simulink model "feed_system_harness_combined"  (R2025b)
settings: Solver=ode23t  StartTime=0  StopTime=8  RelTol=1e-3
undefined symbols (not defined in the file): eregValveDelay, fuelMdot, fuelRho, fuelSetpoint, KcFuel, Kp1Fuel, Kp2Fuel, KpRampTimeFuel, mainValveTime, modelName, OFRatio, T_prop_n2
libraries: fl_lib x11, nesl_utility x9, simulink x4
(part 2 of 2)

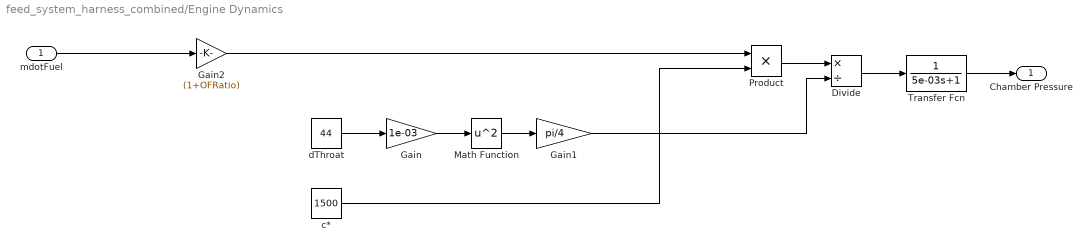
== system feed_system_harness_combined/Engine Dynamics ==
  mdotFuel : Inport
  Divide : Product  Inputs=*/
  Gain : Gain  Gain=1e-03
  Gain1 : Gain  Gain=pi/4
  Gain2 : Gain  Gain=(1+OFRatio)
  Math Function : Math  Operator=square
  Product : Product
  Transfer Fcn : TransferFcn  Denominator=[5e-03 1]
  c* : Constant  Value=1500
  dThroat : Constant  Value=44
  Chamber Pressure : Outport
  wires:
  dThroat/1 -> Gain/1
  Gain/1 -> Math Function/1
  Math Function/1 -> Gain1/1
  c*/1 -> Product/2
  Product/1 -> Divide/1
  Gain1/1 -> Divide/2
  Divide/1 -> Transfer Fcn/1
  Transfer Fcn/1 -> Chamber Pressure/1
  mdotFuel/1 -> Gain2/1
  Gain2/1 -> Product/1

== matlab function feed_system_harness_combined/FeedBack Command ==
  data: propPressure input; propSetpoint input; valveAngle output; nd_error output; Kp input
function [valveAngle, nd_error] = eregControl(propPressure, propSetpoint, Kp)
nd_error = (1 - propPressure/propSetpoint); %Non dimensional error
theta = nd_error * Kp;  %In degrees

valveAngle = deg2rad(theta);

== matlab function feed_system_harness_combined/FeedForwardCommand Fuel ==
  data: n2Pressure input; valveAngle output; CdA_measured output; CdACorrectionFactor input; CdAArray input; mdotProp input; rhoProp input; CdA output
function [valveAngle, CdA_measured, CdA] = feedForwardAngle(n2Pressure, CdACorrectionFactor, CdAArray, mdotProp, rhoProp)
    % Required effective flow area
    CdA_measured = (mdotProp / rhoProp) * 1/sqrt(max(0,n2Pressure)) * 0.673;
    CdA = CdA_measured * CdACorrectionFactor;
% Ball valve opening angle [deg]
    thetaArray = [0, 10, 20, 30, 40, 50, 60, 70, 80, 90];
% Approximate effective CdA for 6 mm bore ball valve [m^2]
    theta = 0;

    % Clamp
    if CdA <= CdAArray(1)

        theta = thetaArray(1);

    elseif CdA >= CdAArray(end)

        theta = thetaArray(end);

    else

        % Linear interpolation between LUT points
        for i = 1:length(CdAArray)-1

            if CdA >= CdAArray(i) && CdA <= CdAArray(i+1)

                theta = thetaArray(i) + ...
                    ((CdA - CdAArray(i)) / ...
                    (CdAArray(i+1) - CdAArray(i))) * ...
                    (thetaArray(i+1) - thetaArray(i));

                break;

            end

        end

    end

    % Output angle in radians
    valveAngle = deg2rad(theta);

end

== matlab function feed_system_harness_combined/CdA Robustness Function ==
  data: array output; shiftBool input; shiftIdx input; scaleFactor input
function array = CdAArray(shiftBool, shiftIdx, scaleFactor)
array   = [0, 0, 0, 4.0e-6, 12.7e-6, 15.2e-6, 17.1e-6, 18.6e-6, 19.5e-6, 19.8e-6];
array = array * scaleFactor;
if shiftBool == true
    array = shiftArray(array, shiftIdx);
end

end

function shifted = shiftArray(array, n)
    % Shifts array by n positions.
    %   n > 0: shifts forward (right), padding the start with the first value
    %   n < 0: shifts backward (left), padding the end with the last value
    %   n = 0: returns array unchanged

    N = numel(array);
    shifted = zeros(size(array));

    if n >= 0
        n = min(n, N);
        shifted(1:n) = array(1);                  % pad start with first value
        shifted(n+1:end) = array(1:N-n);
    else
        n = min(-n, N);
        shifted(1:N-n) = array(n+1:end);
        shifted(N-n+1:end) = array(end);           % pad end with last value
    end
end
